simulink model "classicrelay"  (R2021b)
settings: Solver=FixedStepAuto  StartTime=0.0  StopTime=500  FixedStep=0.2  RelTol=1e-3
undefined symbols (not defined in the file or in its folder): relayBut
settings Model: Creator=ismt  LastModifiedBy=ismt

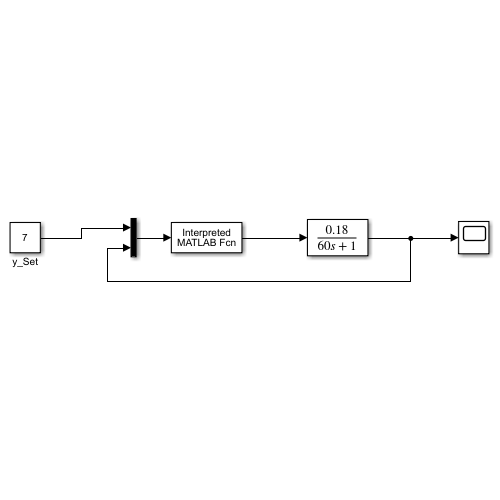
[thumbnail: Simulink's stored preview of the top-level diagram]
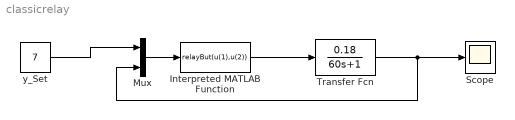
== system classicrelay ==
  Interpreted MATLAB Function : MATLABFcn  MATLABFcn=relayBut(u(1),u(2))
  Mux : Mux  Inputs=2
  Scope : Scope
  Transfer Fcn : TransferFcn  Numerator=[0.18]  Denominator=[60 1]
  y_Set : Constant  Value=7
  wires:
  Interpreted MATLAB Function/1 -> Transfer Fcn/1
  Transfer Fcn/1 -> Mux/2, Scope/1
  Mux/1 -> Interpreted MATLAB Function/1
  y_Set/1 -> Mux/1
